simulink model "kalman_tries"  (R2019a)
settings: Solver=VariableStepAuto  StartTime=0.0  StopTime=100.0  RelTol=1e-3
undefined symbols (not defined in the file or in its folder): DiscIntNeverNeededParam, Kalman_1, Kalman_2
libraries: simulink x4
settings Model: Creator=Gaming  LastModifiedBy=User

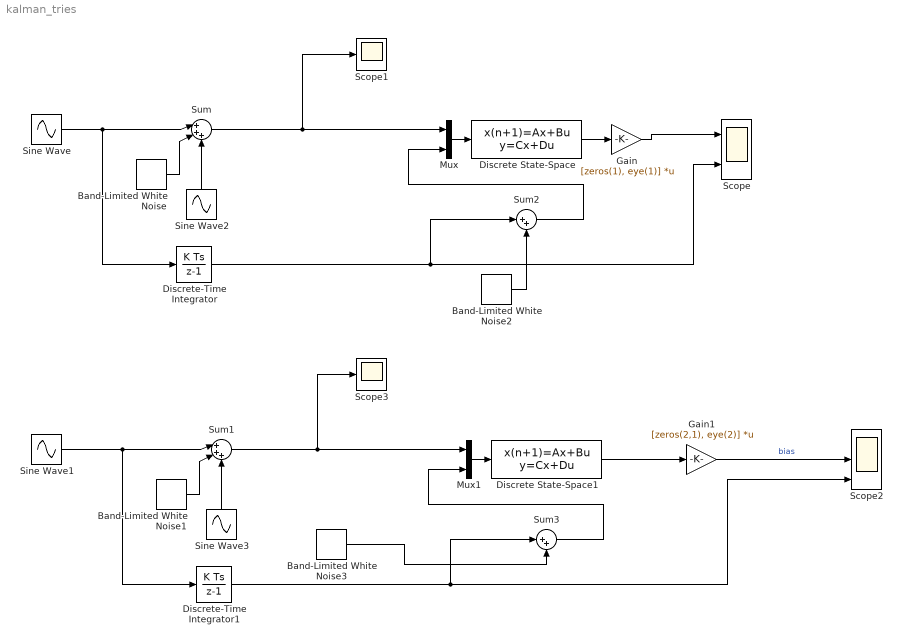
== system kalman_tries ==
  Band-Limited White Noise{,1..3} (4 alike) : simulink/Sources/Band-Limited White Noise  Cov=[0.0001]  Ts=0.1  seed=[23341]
  Discrete State-Space : DiscreteStateSpace  A=Kalman_1.sys.A  B=Kalman_1.sys.B  C=Kalman_1.sys.C  D=Kalman_1.sys.D  SampleTime=-1
  Discrete State-Space1 : DiscreteStateSpace  A=Kalman_2.sys.A  B=Kalman_2.sys.B  C=Kalman_2.sys.C  D=Kalman_2.sys.D  SampleTime=-1
  Discrete-Time Integrator : DiscreteIntegrator  SampleTime=-1  ICPrevOutput=DiscIntNeverNeededParam  ICPrevScaledInput=DiscIntNeverNeededParam
  Discrete-Time Integrator1 : DiscreteIntegrator  SampleTime=-1  ICPrevOutput=DiscIntNeverNeededParam  ICPrevScaledInput=DiscIntNeverNeededParam
  Gain : Gain  Gain=[zeros(1), eye(1)]  Multiplication=Matrix(K*u)
  Gain1 : Gain  Gain=[zeros(2,1), eye(2)]  Multiplication=Matrix(K*u)
  Mux : Mux  Inputs=2
  Mux1 : Mux  Inputs=2
  Scope : Scope  NumInputPorts=2
  Scope1 : Scope
  Scope2 : Scope  NumInputPorts=3
  Scope3 : Scope
  Sine Wave : Sin  SineType=Sample based  Amplitude=0  Samples=100  SampleTime=0.1
  Sine Wave1 : Sin  SineType=Sample based  Amplitude=0  Samples=100  SampleTime=0.1
  Sine Wave2 : Sin  SineType=Sample based  Amplitude=0  Bias=1  Samples=100  SampleTime=0.1
  Sine Wave3 : Sin  SineType=Sample based  Amplitude=0  Bias=1  Samples=100  SampleTime=0.1
  Sum : Sum  Inputs=|+++
  Sum1 : Sum  Inputs=|+++
  Sum2 : Sum  Inputs=|++
  Sum3 : Sum  Inputs=|++
  wires:
  Sine Wave/1 -> Discrete-Time Integrator/1, Sum/1
  Sum/1 -> Mux/1, Scope1/1
  Discrete-Time Integrator/1 -> Scope/2, Sum2/1
  Sine Wave2/1 -> Sum/3
  Sum2/1 -> Mux/2
  Band-Limited White Noise2/1 -> Sum2/2
  Band-Limited White Noise/1 -> Sum/2
  Discrete State-Space/1 -> Gain/1
  Mux/1 -> Discrete State-Space/1
  Band-Limited White Noise3/1 -> Sum3/2
  Sine Wave1/1 -> Discrete-Time Integrator1/1, Sum1/1
  Mux1/1 -> Discrete State-Space1/1
  Band-Limited White Noise1/1 -> Sum1/2
  Sum3/1 -> Mux1/2
  Gain1/1 -> Scope2/2  "bias"
  Sum1/1 -> Mux1/1, Scope3/1
  Discrete-Time Integrator1/1 -> Scope2/3, Sum3/1
  Sine Wave3/1 -> Sum1/3
  Gain/1 -> Scope/1
  Discrete State-Space1/1 -> Gain1/1
